simulink model "DSPequivalent_noMS"  (R2018b)
settings: Solver=ode5  StartTime=0.0  StopTime=MAX_data_count*Tpwm/2  FixedStep=Tsim  RelTol=1e-3
values from neighbouring files (symbols this model uses):
  alfa = 0.17    [init_DSPeq.m]
  beta = exp(-Ts/(R*C))    [init_DSPeq.m]
  C = 110e-9    (= 1.1e-07)    [init_DSPeq.m]
  E = 3.3    [init_DSPeq.m]    (also in init_DSPeq_FOC.m = 520; init_DSPeq_IM.m = 650)
  Ki = 0.2/ur    (= 0.05)    [init_DSPeq.m]    (also in init_DSPeq_FOC.m = wc*Kp/(tan(-pi/2+pm+2*atan(wc*Ts/4)+atan(wc*L/R))))
  Kp = 1.8    [init_DSPeq.m]    (also in init_DSPeq_FOC.m = R*sqrt(1+(wc*L/R)^2))
  Nos = 16    [init_DSPeq.m]    (also in init_DSPeq_FOC.m; init_DSPeq_IM.m)
  OVERSAMPLING = 1    [init_DSPeq.m]    (also in init_DSPeq_FOC.m; init_DSPeq_IM.m; raw_plot.m)
  PWM_TBPRD = 4992    [init_DSPeq.m]    (also in init_DSPeq_FOC.m; init_DSPeq_IM.m; paramSet.m)
  R = 9.92e3    (= 9920)    [init_DSPeq.m]    (also in init_DSPeq_FOC.m = 0.47)
  Rp = 1000e3    (= 1000000)    [init_DSPeq.m]
  Rs = 10    [init_DSPeq.m]    (also in init_DSPeq_IM.m = 13.12)
  Tadc = Tpwm/Nos    (= 6.24e-06)    [init_DSPeq.m]    (also in init_DSPeq_FOC.m; init_DSPeq_IM.m)
  Tpwm = 2*PWM_TBPRD/ftbclk    (= 9.984e-05)    [init_DSPeq.m]    (also in init_DSPeq_FOC.m; init_DSPeq_IM.m; paramSet.m)
  Ts = Tpwm/ur    (= 2.496e-05)    [init_DSPeq.m]    (also in init_DSPeq_FOC.m = 1.248e-05; init_DSPeq_IM.m = 4.992e-05; paramSet.m = 4.992e-05; step_prikaz.m = Ts/1000)
  Ttbclk = 1/ftbclk    (= 1e-08)    [init_DSPeq.m]    (also in init_DSPeq_FOC.m; init_DSPeq_IM.m; paramSet.m)
  ur = 4    [init_DSPeq.m]    (also in init_DSPeq_FOC.m = 8; init_DSPeq_IM.m = 2; paramSet.m = 2; raw_plot.m = 2)
  Vref1 = 0    [init_DSPeq.m]
  Vref2 = 0.5    [init_DSPeq.m]
libraries: simulink x6, simulink_extras x1
settings Model: Creator=ruzic  LastModifiedBy=ruzic

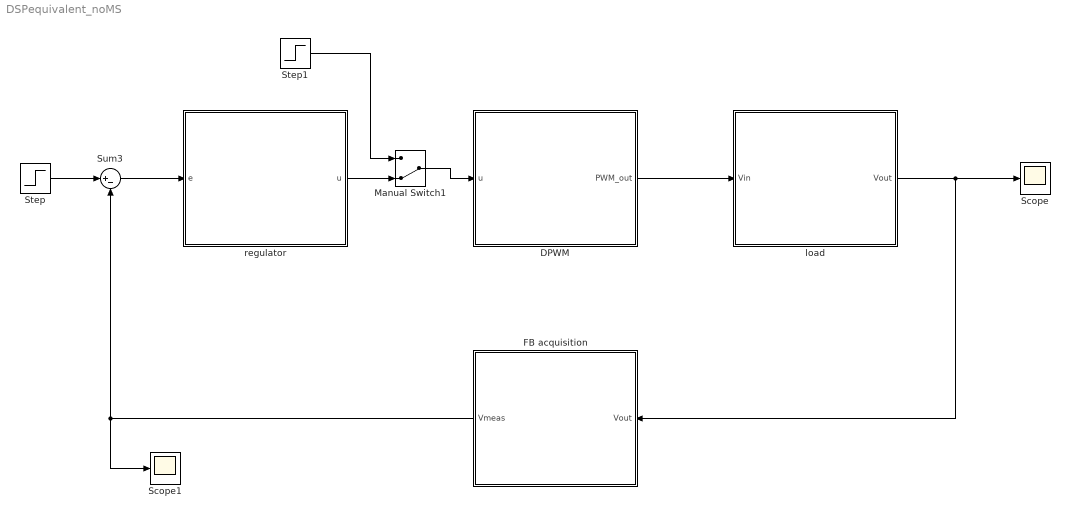
== system DSPequivalent_noMS ==
  DPWM : Subsystem
  FB acquisition : Subsystem
  Manual Switch1 : ManualSwitch  CurrentSetting=0
  Scope : Scope
  Scope1 : Scope
  Step : Step  Time=Tpwm/ur  Before=Vref1  After=Vref2  SampleTime=Ts
  Step1 : Step  Time=0  After=E/2  SampleTime=Ts
  Sum3 : Sum  Inputs=|+-
  load : Subsystem
  regulator : Subsystem
  wires:
  Sum3/1 -> regulator/1(e)
  Step/1 -> Sum3/1
  DPWM/1(PWM_out) -> load/1(Vin)
  load/1(Vout) -> FB acquisition/1(Vout), Scope/1
  FB acquisition/1("Vmeas ") -> Sum3/2, Scope1/1
  regulator/1(u) -> Manual Switch1/2
  Manual Switch1/1 -> DPWM/1(u)
  Step1/1 -> Manual Switch1/1

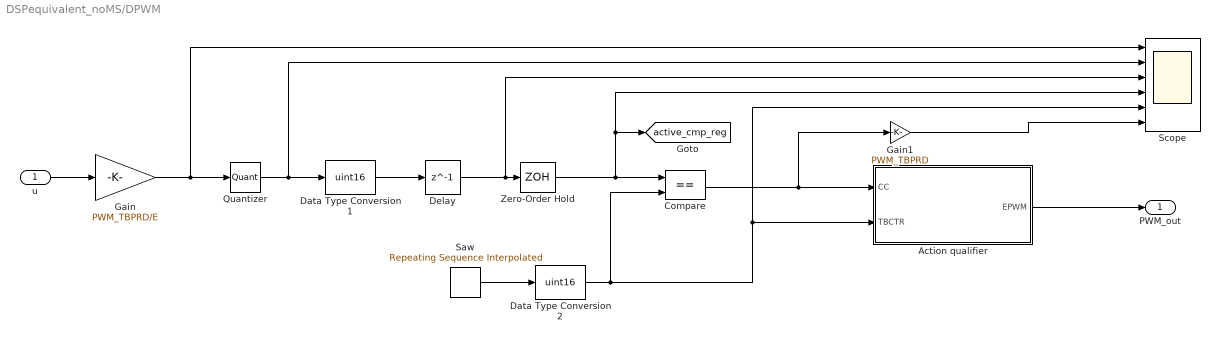
== system DSPequivalent_noMS/DPWM ==
  u : Inport
  Action qualifier : Subsystem
  Compare : RelationalOperator  Operator===  OutDataTypeStr=boolean  RndMeth=Nearest  InputSameDT=on
  Data Type Conversion1 : DataTypeConversion  OutDataTypeStr=uint16  ConvertRealWorld=Stored Integer (SI)  RndMeth=Round
  Data Type Conversion2 : DataTypeConversion  OutDataTypeStr=uint16  ConvertRealWorld=Stored Integer (SI)  RndMeth=Round
  Delay : Delay  DelayLength=1  SampleTime=Ts
  Gain : Gain  Gain=PWM_TBPRD/E
  Gain1 : Gain  Gain=PWM_TBPRD
  Quantizer : Quantizer  QuantizationInterval=1
  Saw : simulink/Sources/Repeating Sequence Interpolated  OutValues=[0 PWM_TBPRD 1].'  TimeValues=[0 Tpwm/2 (Tpwm-Ttbclk)].'  LookUpMeth=Interpolation-Use End Values  tsamp=Ttbclk  OutMin=[]  OutMax=[]  OutDataTypeStr=double  OutputDataTypeScalingMode=double  OutDataType=fixdt(0,8)  OutScaling=2^-10
  Scope : Scope  NumInputPorts=6
  Zero-Order Hold : ZeroOrderHold  SampleTime=-1
  PWM_out : Outport
  tag scope: active_cmp_reg=global
  wires:
  u/1 -> Gain/1
  Gain/1 -> Scope/1, Quantizer/1
  Quantizer/1 -> Data Type Conversion1/1, Scope/2
  Delay/1 -> Scope/3, Zero-Order Hold/1
  Saw/1 -> Data Type Conversion2/1
  Zero-Order Hold/1 -> Compare/1, [active_cmp_reg], Scope/4
  Data Type Conversion1/1 -> Delay/1
  Data Type Conversion2/1 -> Compare/2, Scope/5, Action qualifier/2(TBCTR)
  Compare/1 -> Gain1/1, Action qualifier/1(CC)
  Gain1/1 -> Scope/6
  Action qualifier/1(EPWM) -> PWM_out/1

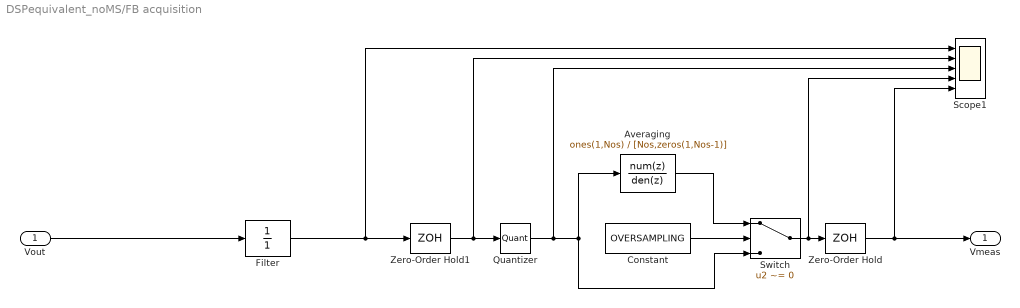
== system DSPequivalent_noMS/FB acquisition ==
  Vout : Inport
  Averaging : DiscreteTransferFcn  Numerator=ones(1,Nos)  Denominator=[Nos,zeros(1,Nos-1)]
  Constant : Constant  Value=OVERSAMPLING
  Filter : TransferFcn  Denominator=[1]
  Quantizer : Quantizer  QuantizationInterval=3/(2^12-1)
  Scope1 : Scope  NumInputPorts=5
  Switch : Switch  Criteria=u2 ~= 0
  Zero-Order Hold : ZeroOrderHold  SampleTime=Ts
  Zero-Order Hold1 : ZeroOrderHold  SampleTime=Tadc
  "Vmeas " : Outport
  wires:
  Zero-Order Hold1/1 -> Quantizer/1, Scope1/2
  Filter/1 -> Zero-Order Hold1/1, Scope1/1
  Vout/1 -> Filter/1
  Zero-Order Hold/1 -> Scope1/5, "Vmeas "/1
  Constant/1 -> Switch/2
  Averaging/1 -> Switch/1
  Quantizer/1 -> Switch/3, Averaging/1, Scope1/3
  Switch/1 -> Scope1/4, Zero-Order Hold/1

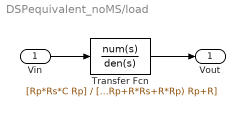
== system DSPequivalent_noMS/load ==
  Vin : Inport
  Transfer Fcn : TransferFcn  Numerator=[Rp*Rs*C Rp]  Denominator=[C*(Rs*Rp+R*Rs+R*Rp) Rp+R]
  Vout : Outport
  wires:
  Vin/1 -> Transfer Fcn/1
  Transfer Fcn/1 -> Vout/1

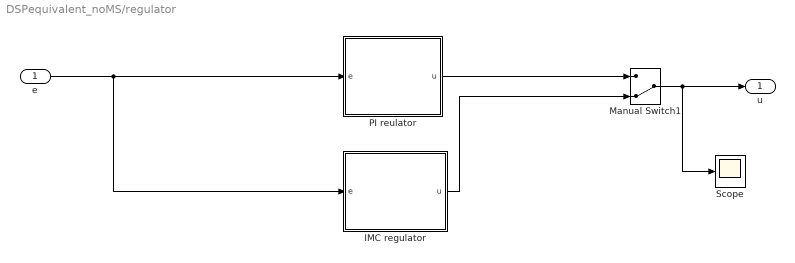
== system DSPequivalent_noMS/regulator ==
  e : Inport
  IMC regulator : Subsystem
  Manual Switch1 : ManualSwitch  CurrentSetting=0
  PI reulator : Subsystem
  Scope : Scope
  u : Outport
  wires:
  e/1 -> IMC regulator/1(e), PI reulator/1(e)
  Manual Switch1/1 -> Scope/1, u/1
  PI reulator/1(u) -> Manual Switch1/1
  IMC regulator/1(u) -> Manual Switch1/2

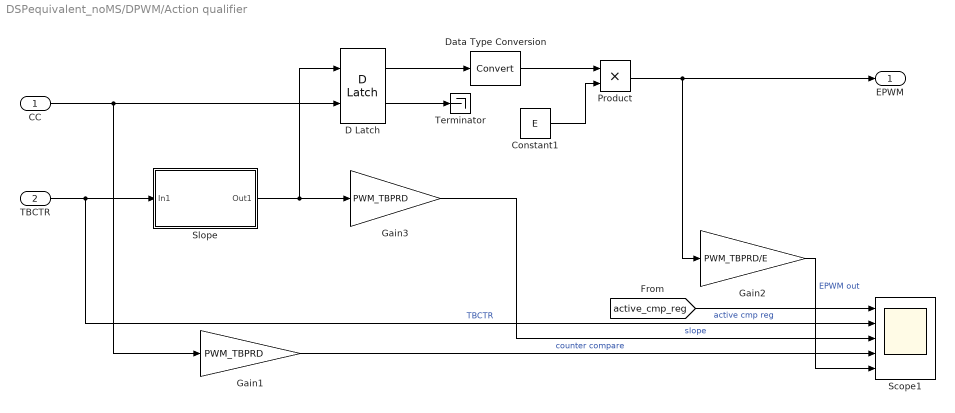
== system DSPequivalent_noMS/DPWM/Action qualifier ==
  CC : Inport
  TBCTR : Inport  Port=2
  Constant1 : Constant  Value=E
  D Latch : simulink_extras/Flip Flops/D Latch
      settings: SourceProductName=Simulink  SourceProductBaseCode=SL
  Data Type Conversion : DataTypeConversion
  Gain1 : Gain  Gain=PWM_TBPRD
  Gain2 : Gain  Gain=PWM_TBPRD/E
  Gain3 : Gain  Gain=PWM_TBPRD
  Product : Product
  Scope1 : Scope  NumInputPorts=5
  Slope : Subsystem
  Terminator : Terminator
  EPWM : Outport
  wires:
  Gain3/1 -> Scope1/3  "slope"
  D Latch/2 -> Terminator/1
  Slope/1(Out1) -> D Latch/1, Gain3/1
  Product/1 -> EPWM/1, Gain2/1
  CC/1 -> D Latch/2, Gain1/1
  Data Type Conversion/1 -> Product/1
  [active_cmp_reg] -> Scope1/1  "active cmp reg"
  Gain2/1 -> Scope1/5  "EPWM out"
  Constant1/1 -> Product/2
  Gain1/1 -> Scope1/4  "counter compare"
  D Latch/1 -> Data Type Conversion/1
  TBCTR/1 -> Scope1/2, Slope/1(In1)  "TBCTR"

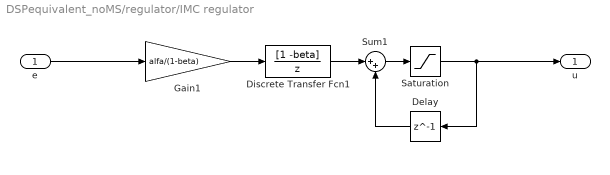
== system DSPequivalent_noMS/regulator/IMC regulator ==
  e : Inport
  Delay : Delay  DelayLength=1
  Discrete Transfer Fcn1 : DiscreteTransferFcn  Numerator=[1 -beta]  Denominator=[1 0]  SampleTime=Ts
  Gain1 : Gain  Gain=alfa/(1-beta)
  Saturation : Saturate  UpperLimit=E  LowerLimit=0
  Sum1 : Sum  Inputs=|++
  u : Outport
  wires:
  e/1 -> Gain1/1
  Sum1/1 -> Saturation/1
  Delay/1 -> Sum1/2
  Discrete Transfer Fcn1/1 -> Sum1/1
  Gain1/1 -> Discrete Transfer Fcn1/1
  Saturation/1 -> u/1, Delay/1

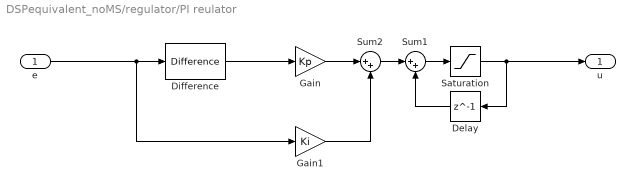
== system DSPequivalent_noMS/regulator/PI reulator ==
  e : Inport
  Delay : Delay  DelayLength=1
  Difference : simulink/Discrete/Difference  ICPrevInput=0.0  OutMin=[]  OutMax=[]  OutDataType=fixdt(1, 16)  OutScaling=2^-10  DoSatur=off
  Gain : Gain  Gain=Kp
  Gain1 : Gain  Gain=Ki
  Saturation : Saturate  UpperLimit=E  LowerLimit=0
  Sum1 : Sum  Inputs=|++
  Sum2 : Sum  Inputs=|++
  u : Outport
  wires:
  Saturation/1 -> u/1, Delay/1
  Gain/1 -> Sum2/1
  e/1 -> Gain1/1, Difference/1
  Delay/1 -> Sum1/2
  Sum1/1 -> Saturation/1
  Sum2/1 -> Sum1/1
  Gain1/1 -> Sum2/2
  Difference/1 -> Gain/1

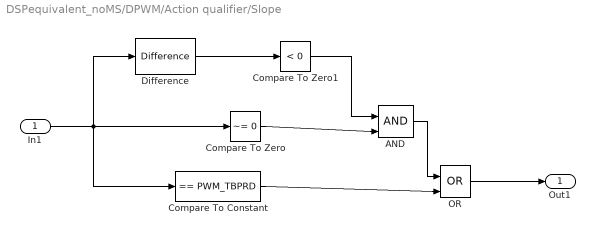
== system DSPequivalent_noMS/DPWM/Action qualifier/Slope ==
  In1 : Inport
  AND : Logic  IconShape=distinctive  AllPortsSameDT=off  OutDataTypeStr=boolean
  Compare To Constant : simulink/Logic and Bit Operations/Compare To Constant  relop===  const=PWM_TBPRD  OutDataTypeStr=boolean
  Compare To Zero : simulink/Logic and Bit Operations/Compare To Zero  relop=~=  OutDataTypeStr=boolean
  Compare To Zero1 : simulink/Logic and Bit Operations/Compare To Zero  relop=<  OutDataTypeStr=boolean
  Difference : simulink/Discrete/Difference  ICPrevInput=0  OutMin=[]  OutMax=[]  OutDataTypeStr=int16  OutputDataTypeScalingMode=int16  OutDataType=fixdt(1, 16)  OutScaling=2^-10  DoSatur=off
  OR : Logic  Operator=OR  IconShape=distinctive  AllPortsSameDT=off  OutDataTypeStr=boolean
  Out1 : Outport
  wires:
  In1/1 -> Difference/1, Compare To Constant/1, Compare To Zero/1
  AND/1 -> OR/1
  Compare To Zero1/1 -> AND/1
  Compare To Constant/1 -> OR/2
  Difference/1 -> Compare To Zero1/1
  OR/1 -> Out1/1
  Compare To Zero/1 -> AND/2
